simulink model "pid_pi_pd_basic"  (R2021a)
settings: Solver=VariableStepAuto  StartTime=0.0  StopTime=10.0  RelTol=1e-3
libraries: spspowerguiLib x1
settings Model: Creator=LENOVO  LastModifiedBy=LENOVO

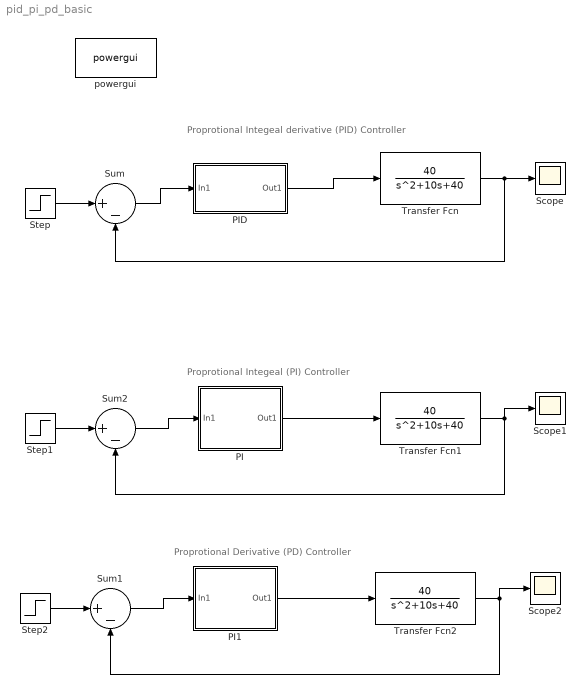
== system pid_pi_pd_basic ==
  note: Proprotional Integeal derivative (PID) Controller
  note: Proprotional Integeal (PI) Controller
  note: Proprotional Derivative (PD) Controller
  PI : Subsystem
  PI1 : Subsystem
  PID : Subsystem
  Scope : Scope
  Scope1 : Scope
  Scope2 : Scope
  Step : Step  Time=0  SampleTime=0
  Step1 : Step  Time=0  SampleTime=0
  Step2 : Step  Time=0  SampleTime=0
  Sum : Sum  Inputs=|+-
  Sum1 : Sum  Inputs=|+-
  Sum2 : Sum  Inputs=|+-
  Transfer Fcn : TransferFcn  Numerator=[40]  Denominator=[1 10 40]
  Transfer Fcn1 : TransferFcn  Numerator=[40]  Denominator=[1 10 40]
  Transfer Fcn2 : TransferFcn  Numerator=[40]  Denominator=[1 10 40]
  powergui : spspowerguiLib/powergui  Priority=1  SimulationMode=Continuous  SampleTime=50e-6  frequency=60  Iterations=50  frequencyindice=60  Pbase=100e6  ErrMax=1e-4  UnitsV=kV  UnitsW=MW  buscounter=0  FunctionMessages=off  echomessages=off  EnableUseOfTLC=off  CurrentSourceSwitches=off  DisableSnubberDevices=off  DisableRonSwitches=off  DisableVfSwitches=off  DisplayEquations=off  AutomaticDiscreteSolvers=off  SolverType=Tustin/Backward Euler (TBE)  Interpol=off  ExternalGateDelay=off  methode=off  Ts=100  x0status=blocks  SPID=on  SwTol=0  HookPort=off  NonlinearTolerance=1e-4  nMaxIteration=100  ContinueOnMaxIteration=off  RestoreLinks=warning  ResistiveCurrentMeasurement=off  Frange=[0:2:500]  Ylog=off  Xlog=on  ShowGrid=off  save=off  variable=ZData  structure=0  ZoomFFT=off  StartTime=0.0  cycles=1  DisplayStyle=1  fundamental=60  FreqAxis=off  MaxFrequency=1000  frequencyindicesteady=1  RmsSteady=1  display=off
  wires:
  Step/1 -> Sum/1
  Transfer Fcn/1 -> Sum/2, Scope/1
  Transfer Fcn1/1 -> Scope1/1, Sum2/2
  Step1/1 -> Sum2/1
  Sum/1 -> PID/1(In1)
  PID/1(Out1) -> Transfer Fcn/1
  Sum2/1 -> PI/1(In1)
  PI/1(Out1) -> Transfer Fcn1/1
  PI1/1(Out1) -> Transfer Fcn2/1
  Sum1/1 -> PI1/1(In1)
  Step2/1 -> Sum1/1
  Transfer Fcn2/1 -> Sum1/2, Scope2/1

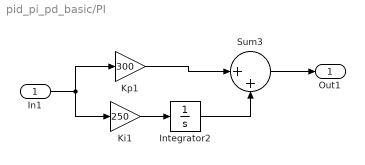
== system pid_pi_pd_basic/PI ==
  In1 : Inport
  Integrator2 : Integrator
  Ki1 : Gain  Gain=250
  Kp1 : Gain  Gain=300
  Sum3 : Sum  Inputs=|++
  Out1 : Outport
  wires:
  In1/1 -> Ki1/1, Kp1/1
  Integrator2/1 -> Sum3/2
  Ki1/1 -> Integrator2/1
  Kp1/1 -> Sum3/1
  Sum3/1 -> Out1/1

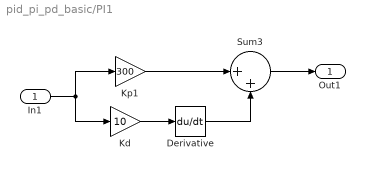
== system pid_pi_pd_basic/PI1 ==
  In1 : Inport
  Derivative : Derivative
  Kd : Gain  Gain=10
  Kp1 : Gain  Gain=300
  Sum3 : Sum  Inputs=|++
  Out1 : Outport
  wires:
  Sum3/1 -> Out1/1
  Kp1/1 -> Sum3/1
  Kd/1 -> Derivative/1
  Derivative/1 -> Sum3/2
  In1/1 -> Kp1/1, Kd/1

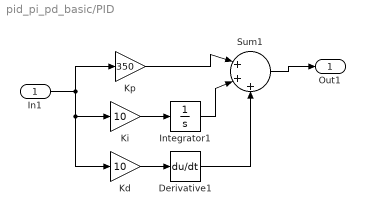
== system pid_pi_pd_basic/PID ==
  In1 : Inport
  Derivative1 : Derivative
  Integrator1 : Integrator
  Kd : Gain  Gain=10
  Ki : Gain  Gain=10
  Kp : Gain  Gain=350
  Sum1 : Sum  Inputs=|+++
  Out1 : Outport
  wires:
  Derivative1/1 -> Sum1/3
  Ki/1 -> Integrator1/1
  Sum1/1 -> Out1/1
  In1/1 -> Kp/1, Kd/1, Ki/1
  Kd/1 -> Derivative1/1
  Kp/1 -> Sum1/1
  Integrator1/1 -> Sum1/2
